simulink model "un5"  (R2021b)
settings: Solver=FixedStepAuto  StartTime=0.0  StopTime=0.5  FixedStep=0.001  RelTol=1e-3
libraries: simulink x1
settings Model: Creator=dkole  LastModifiedBy=Ivan
settings SolverCC: AlgebraicLoopSolver=TrustRegion
settings DebuggingCC: SFMachineParentedDataDiag=warning

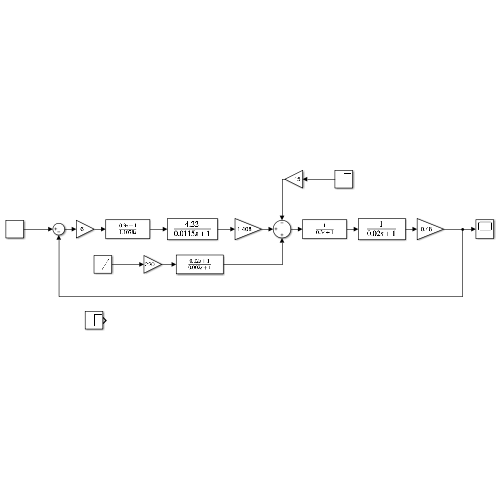
[thumbnail: Simulink's stored preview of the top-level diagram]
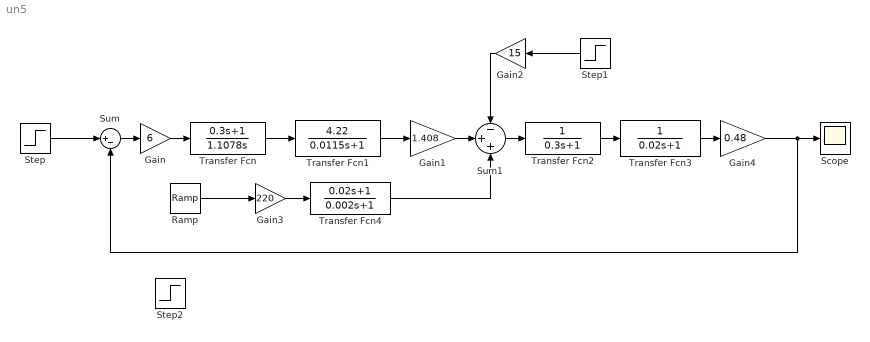
== system un5 ==
  Gain : Gain  Gain=6
  Gain1 : Gain  Gain=1.408
  Gain2 : Gain  Gain=15
  Gain3 : Gain  Gain=220
  Gain4 : Gain  Gain=0.48
  Ramp : simulink/Sources/Ramp  slope=0  start=0  InitialOutput=0
  Scope : Scope
  Step : Step  Time=0  After=500  SampleTime=0
  Step1 : Step  Time=0  After=0  SampleTime=0
  Step2 : Step  Time=0  After=3  SampleTime=0
  Sum : Sum  Inputs=|+-
  Sum1 : Sum  Inputs=-++
  Transfer Fcn : TransferFcn  Numerator=[0.3 1]  Denominator=[1.1078 0]
  Transfer Fcn1 : TransferFcn  Numerator=[4.22]  Denominator=[0.0115 1]
  Transfer Fcn2 : TransferFcn  Denominator=[0.3 1]
  Transfer Fcn3 : TransferFcn  Denominator=[0.02 1]
  Transfer Fcn4 : TransferFcn  Numerator=[0.02 1]  Denominator=[0.002 1]
  wires:
  Transfer Fcn/1 -> Transfer Fcn1/1
  Sum1/1 -> Transfer Fcn2/1
  Transfer Fcn1/1 -> Gain1/1
  Gain2/1 -> Sum1/1
  Transfer Fcn2/1 -> Transfer Fcn3/1
  Gain3/1 -> Transfer Fcn4/1
  Transfer Fcn4/1 -> Sum1/3
  Transfer Fcn3/1 -> Gain4/1
  Gain/1 -> Transfer Fcn/1
  Sum/1 -> Gain/1
  Step/1 -> Sum/1
  Gain1/1 -> Sum1/2
  Gain4/1 -> Sum/2, Scope/1
  Step1/1 -> Gain2/1
  Ramp/1 -> Gain3/1
